simulink model "RLC_"  (R2021a)
settings: Solver=VariableStepAuto  StartTime=0.0  StopTime=0.18  RelTol=1e-3
values from neighbouring files (symbols this model uses):
  C = 0.0001    [RLC.m]
  L = 0.001    [RLC.m]
  R = 200    [RLC.m]
settings Model: Creator=melan  LastModifiedBy=melan

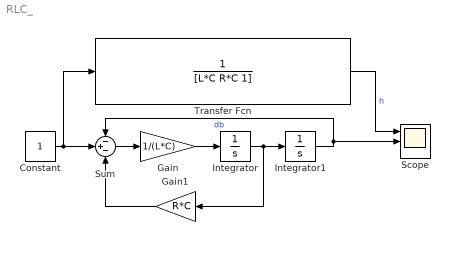
== system RLC_ ==
  Constant : Constant
  Gain : Gain  Gain=1/(L*C)
  Gain1 : Gain  Gain=R*C
  Integrator : Integrator
  Integrator1 : Integrator
  Scope : Scope  NumInputPorts=3
  Sum : Sum  Inputs=-+-
  Transfer Fcn : TransferFcn  Denominator=[L*C R*C 1]
  wires:
  Gain/1 -> Integrator/1
  Integrator/1 -> Gain1/1, Integrator1/1
  Sum/1 -> Gain/1
  Integrator1/1 -> Sum/1, Scope/2  "db"
  Gain1/1 -> Sum/3
  Constant/1 -> Transfer Fcn/1, Sum/2
  Transfer Fcn/1 -> Scope/1  "h"
